simulink library "PM_BLDC"  (R2024a)
settings: Solver=VariableStepAuto  StartTime=0.0  StopTime=10.0  RelTol=1e-3
undefined symbols (not defined in the file): B, J, Ke, Ls, P, Rs
settings Model: Creator=Mohamed Draz  LastModifiedBy=Mohamed Draz

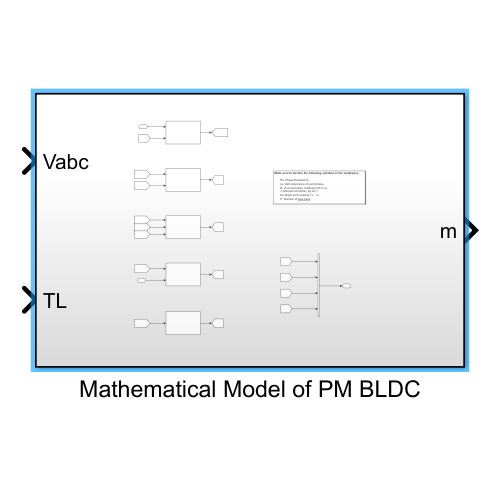
[thumbnail: Simulink's stored preview of the top-level diagram]
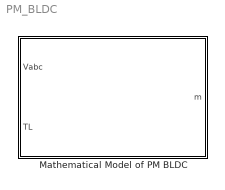
== system PM_BLDC ==
  Mathematical Model of PM BLDC : Subsystem

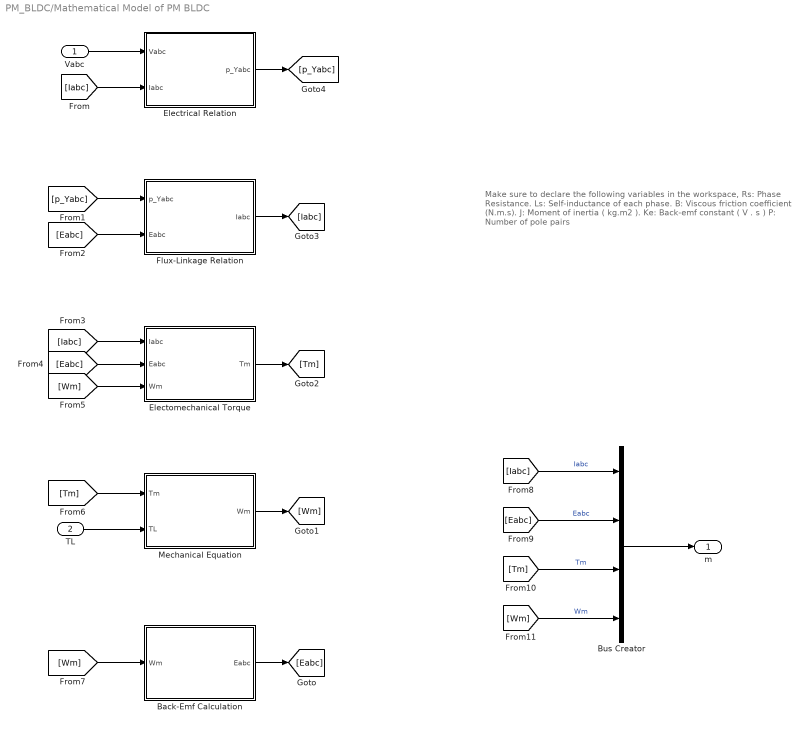
== system PM_BLDC/Mathematical Model of PM BLDC ==
  note: Make sure to declare the following variables in the workspace,
      |
      | Rs: Phase Resistance.
      | Ls: Self-inductance of each phase.
      | B: Viscous friction coefficient (N.m.s).
      | J: Moment of inertia ( kg.m2 ).
      | Ke: Back-emf constant ( V . s )
      | P: Number of pole pairs
  Vabc : Inport
  TL : Inport  Port=2
  Back-Emf Calculation : Subsystem
  Bus Creator : BusCreator  Inputs=4
  Electomechanical Torque : Subsystem
  Electrical Relation : Subsystem
  Flux-Linkage Relation : Subsystem
  Mechanical Equation : Subsystem
  m : Outport
  wires:
  [Wm] -> Back-Emf Calculation/1(Wm)
  [Eabc] -> Electomechanical Torque/2(Eabc)
  Electomechanical Torque/1(Tm) -> [Tm]
  Flux-Linkage Relation/1(Iabc) -> [Iabc]
  [Wm] -> Electomechanical Torque/3(Wm)
  [p_Yabc] -> Flux-Linkage Relation/1(p_Yabc)
  [Eabc] -> Flux-Linkage Relation/2(Eabc)
  [Iabc] -> Electomechanical Torque/1(Iabc)
  [Tm] -> Mechanical Equation/1(Tm)
  Back-Emf Calculation/1(Eabc) -> [Eabc]
  Vabc/1 -> Electrical Relation/1(Vabc)
  [Iabc] -> Electrical Relation/2(Iabc)
  TL/1 -> Mechanical Equation/2(TL)
  Electrical Relation/1(p_Yabc) -> [p_Yabc]
  Mechanical Equation/1(Wm) -> [Wm]
  [Iabc] -> Bus Creator/1  "Iabc"
  [Eabc] -> Bus Creator/2  "Eabc"
  [Tm] -> Bus Creator/3  "Tm"
  [Wm] -> Bus Creator/4  "Wm"
  Bus Creator/1 -> m/1

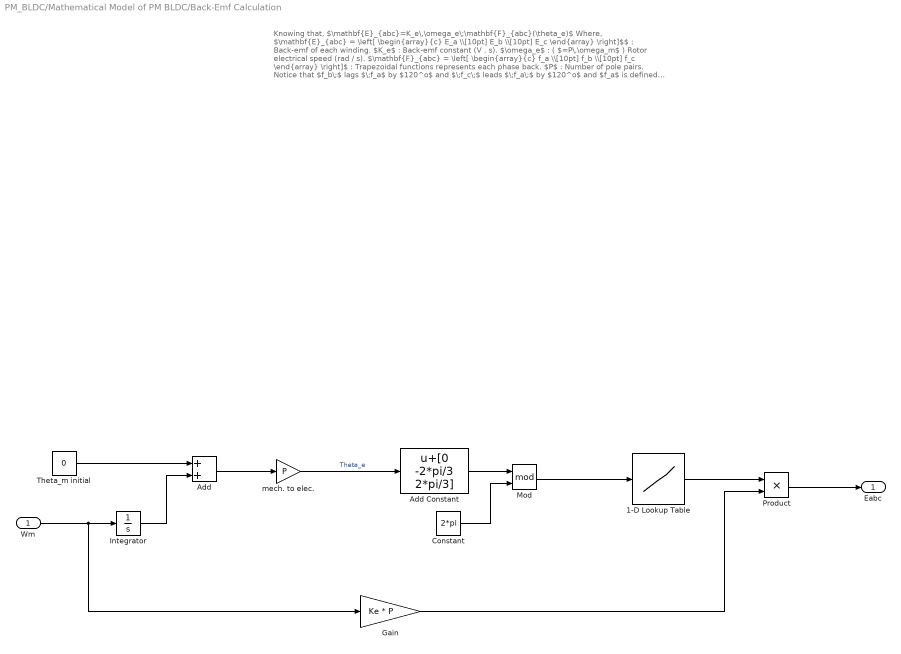
== system PM_BLDC/Mathematical Model of PM BLDC/Back-Emf Calculation ==
  note: Knowing that,
      |
      | $\mathbf{E}_{abc}=K_e\,\omega_e\;\mathbf{F}_{abc}(\theta_e)$
      |
      | Where,
      |
      | $\mathbf{E}_{abc} = \left[ \begin{array}{c} E_a \\[10pt] E_b \\[10pt] E_c \end{array} \right]$$ : Back-emf of each winding.
      |
      | $K_e$ : Back-emf constant (V . s).
      |
      | $\omega_e$ : ( $=P\,\omega_m$ ) Rotor electrical speed (rad / s).
      |
      | $\mathbf{F}_{abc} = \left[ \begin{array}{c} f_a \\[10pt] f_b \\[10pt] f_c \end{array} \right]$ : Trapezoidal functions represents each phase back.
      |
      | $P$ : Number of pole pairs.
      |
      | Notice that $f_b\;$ lags $\;f_a$ by $120^o$ and $\;f_c\;$ leads $\;f_a\;$ by $120^o$
      |
      | and $f_a$ is defined as,
      |
      | $f_a(\theta) = \begin{cases} 1 & 0 < \theta \le \frac{2\pi}{3} \\[6pt] 1 - \frac{6}{\pi}\left(\theta - \frac{2\pi}{3}\right) & \frac{2\pi}{3} < \theta \le \pi \\[6pt] -1 & \pi < \theta \le \frac{5\pi}{3} \\[6pt] -1 + \frac{6}{\pi}\left(\theta - \frac{5\pi}{3}\right) & \frac{5\pi}{3} < \theta \le 2\pi \end{cases}$$
  Wm : Inport
  1-D Lookup Table : Lookup_n-D  NumberOfTableDimensions=1  BreakpointsSpecification=Even spacing  BreakpointsForDimension1=[-5:5]  BreakpointsForDimension1FirstPoint=0  BreakpointsForDimension1Spacing=2*pi/6  Table=[1 1 1 -1 -1 -1 1]  InternalRulePriority=Speed  RndMeth=Simplest
  Add : Sum
  Add Constant : Bias  Bias=[0 -2*pi/3 2*pi/3]  SaturateOnIntegerOverflow=off
  Constant : Constant  Value=2*pi
  Gain : Gain  Gain=Ke * P
  Integrator : Integrator
  Mod : Math  Operator=mod
  Product : Product
  Theta_m initial : Constant  Value=0
  mech. to elec. : Gain  Gain=P
  Eabc : Outport
  wires:
  Add Constant/1 -> Mod/1
  Constant/1 -> Mod/2
  mech. to elec./1 -> Add Constant/1  "Theta_e"
  Theta_m initial/1 -> Add/1
  Mod/1 -> 1-D Lookup Table/1
  Gain/1 -> Product/2
  1-D Lookup Table/1 -> Product/1
  Wm/1 -> Gain/1, Integrator/1
  Product/1 -> Eabc/1
  Add/1 -> mech. to elec./1
  Integrator/1 -> Add/2

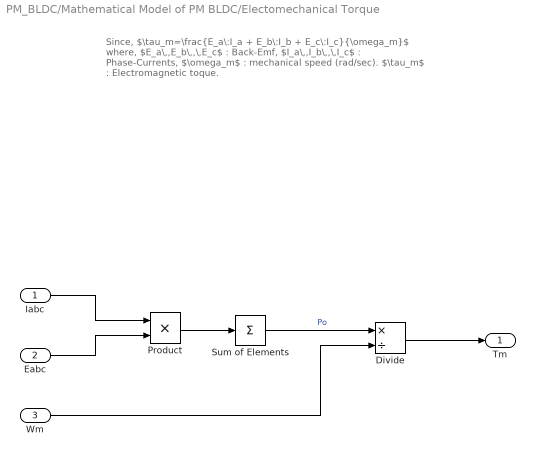
== system PM_BLDC/Mathematical Model of PM BLDC/Electomechanical Torque ==
  note: Since,
      |
      | $\tau_m=\frac{E_a\:I_a + E_b\:I_b + E_c\:I_c}{\omega_m}$
      |
      | where,
      |
      | $E_a\,,E_b\,,\,E_c$ : Back-Emf,
      | $I_a\,,I_b\,,\,I_c$ : Phase-Currents,
      | $\omega_m$ : mechanical speed (rad/sec).
      | $\tau_m$ : Electromagnetic toque.
  Iabc : Inport
  Eabc : Inport  Port=2
  Wm : Inport  Port=3
  Divide : Product  Inputs=*/
  Product : Product
  Sum of Elements : Sum  Inputs=+
  Tm : Outport
  wires:
  Sum of Elements/1 -> Divide/1  "Po"
  Wm/1 -> Divide/2
  Product/1 -> Sum of Elements/1
  Divide/1 -> Tm/1
  Iabc/1 -> Product/1
  Eabc/1 -> Product/2

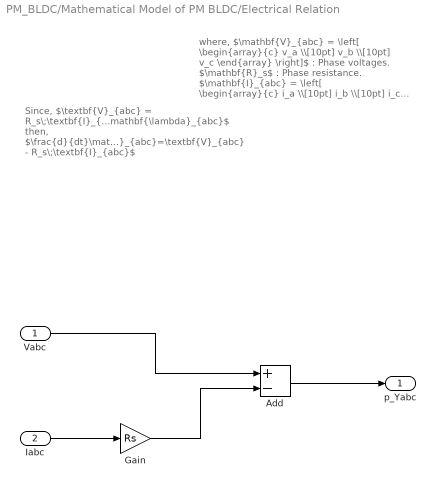
== system PM_BLDC/Mathematical Model of PM BLDC/Electrical Relation ==
  note: Since,
      | $\textbf{V}_{abc} = R_s\;\textbf{I}_{abc}+\frac{d}{dt}\mathbf{\lambda}_{abc}$
      |
      | then,
      | $\frac{d}{dt}\mathbf{\lambda}_{abc}=\textbf{V}_{abc} - R_s\;\textbf{I}_{abc}$
  note: where,
      | $\mathbf{V}_{abc} = \left[ \begin{array}{c} v_a \\[10pt] v_b \\[10pt] v_c \end{array} \right]$ : Phase voltages.
      |
      | $\mathbf{R}_s$ : Phase resistance.
      |
      | $\mathbf{I}_{abc} = \left[ \begin{array}{c} i_a \\[10pt] i_b \\[10pt] i_c \end{array} \right]$ Phase currents
      |
      | $\mathbf{\lambda}_{abc} = \left[ \begin{array}{c} \lambda_a \\[10pt] \lambda_b \\[10pt] \lambda_c \end{array} \right]$ Flux-linkages
  Vabc : Inport
  Iabc : Inport  Port=2
  Add : Sum  Inputs=+-
  Gain : Gain  Gain=Rs
  p_Yabc : Outport
  wires:
  Iabc/1 -> Gain/1
  Add/1 -> p_Yabc/1
  Gain/1 -> Add/2
  Vabc/1 -> Add/1

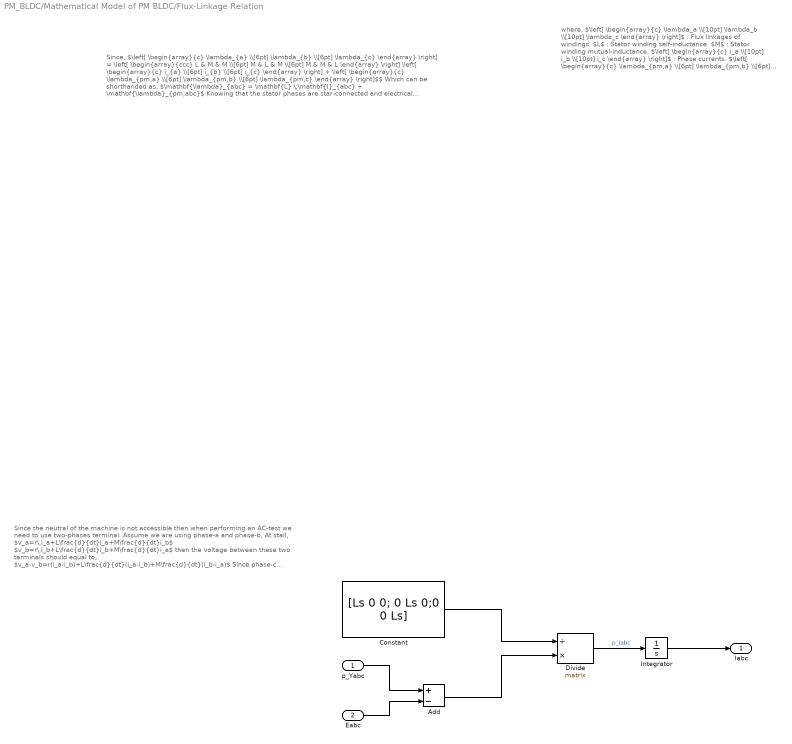
== system PM_BLDC/Mathematical Model of PM BLDC/Flux-Linkage Relation ==
  note: Since,
      |
      | $\left[ \begin{array}{c} \lambda_{a} \\[6pt] \lambda_{b} \\[6pt] \lambda_{c} \end{array} \right] = \left[ \begin{array}{ccc} L & M & M \\[6pt] M & L & M \\[6pt] M & M & L \end{array} \right] \left[ \begin{array}{c} i_{a} \\[6pt] i_{b} \\[6pt] i_{c} \end{array} \right] + \left[ \begin{array}{c} \lambda_{pm,a} \\[6pt] \lambda_{pm,b} \\[6pt] \lambda_{pm,c} \end{array} \right]$$
      |
      | Which can be shorthanded as,
      |
      | $\mathbf{\lambda}_{abc} = \mathbf{L} \;\mathbf{I}_{abc} + \mathbf{\lambda}_{pm,abc}$
      |
      | Knowing that the stator phases are star-connected and electrical parametes are assumed balanced,
      |
      | $i_a+i_b+i_c=0 \rightarrow i_b+i_c=-i_a$
      |
      | thus,
      | $\lambda_a=L\;i_a+M\;i_b+M\;i_c+\lambda_{pm,a}$
      |
      | turns into,
      | $\lambda_a=(L-M)\;i_a+\lambda_{pm,a}$
      |
      | The same could be done to windings b and c. So the original matrix turns into,
      |
      | $\left[ \begin{array}{c} \lambda_{a} \\[6pt] \lambda_{b} \\[6pt] \lambda_{c} \end{array} \right] = \left[ \begin{array}{ccc} L-M & 0 & 0 \\[6pt] 0 & L-M & 0 \\[6pt] 0 & 0 & L-M \end{array} \right] \left[ \begin{array}{c} i_{a} \\[6pt] i_{b} \\[6pt] i_{c} \end{array} \right] + \left[ \begin{array}{c} \lambda_{pm,a} \\[6pt] \lambda_{pm,b} \\[6pt] \lambda_{pm,c} \end{array} \right]$
      |
      | which can be short-handed as,
      |
      | $\mathbf{\lambda}_{abc} = \mathbf{L}_{new} \;\mathbf{I}_{abc} + \mathbf{\lambda}_{pm,abc}$
      |
      | Since $L$ and $M$ are both constants, taking the dervitave of both sides of equation results into,
      |
      | $\frac{d}{dt}\mathbf{\lambda}_{abc} = \mathbf{L}_{new} \;\frac{d}{dt}\mathbf{I}_{abc} + \frac{d}{dt}\mathbf{\lambda}_{pm,abc}$
      |
      | since $\frac{d}{dt}\mathbf{\lambda}_{pm,abc}$ is the the open-circuit voltage of each phase (i.e., Back-emf ) ,
      |
      | $\frac{d}{dt}\mathbf{\lambda}_{abc} = \mathbf{L}_{new} \;\frac{d}{dt}\mathbf{I}_{abc} + \mathbf{E}_{abc}$
      |
      | Finally,
      |
      | $\frac{d}{dt}\mathbf{I}_{abc} = \mathbf{L}_{new}^{-1} \;\left(\frac{d}{dt}\mathbf{\lambda}_{abc}-\mathbf{E}_{abc}\right)$
  note: where,
      |
      | $\left[ \begin{array}{c} \lambda_a \\[10pt] \lambda_b \\[10pt] \lambda_c \end{array} \right]$ : Flux linkages of windings.
      |
      | $L$ : Stator winding self-inductance.
      |
      | $M$ : Stator winding mutual-inductance.
      |
      | $\left[ \begin{array}{c} i_a \\[10pt] i_b \\[10pt] i_c \end{array} \right]$ : Phase currents.
      |
      | $\left[ \begin{array}{c} \lambda_{pm,a} \\[6pt] \lambda_{pm,b} \\[6pt] \lambda_{pm,c} \end{array} \right]$ : Flux-linkages caused by the permanent magent.
  note: Since the neutral of the machine is not accessible then when performing an AC-test we need to use two-phases terminal. Assume we are using phase-a and phase-b,
      |
      | At stall,
      |
      | $v_a=r\,i_a+L\frac{d}{dt}i_a+M\frac{d}{dt}i_b$
      | $v_b=r\,i_b+L\frac{d}{dt}i_b+M\frac{d}{dt}i_a$
      |
      | then the voltage between these two terminals should equal to,
      |
      | $v_a-v_b=r(i_a-i_b)+L\frac{d}{dt}(i_a-i_b)+M\frac{d}{dt}(i_b-i_a)$
      |
      | Since phase-c during this test is open-circuit. then, $i_a=-i_b=i$ . So,
      |
      | $v_a-v_b=2r\,i+2L\frac{d}{dt}i-2M\frac{d}{dt}i$
      | $v_a-v_b=2r\,i+2(L-M)\frac{d}{dt}i$
      |
      | this latest equation reveals that the inductance value measured between two phases during AC test is actually 2(L-M). So the phase-inductance value measured during AC-test mathimatically equals to (L-M).
      |
      | Finally,
      |
      | $L_s=L-M$
  p_Yabc : Inport
  Eabc : Inport  Port=2
  Add : Sum  Inputs=+-
  Constant : Constant  Value=[Ls 0 0; 0 Ls 0;0 0 Ls]  VectorParams1D=off
  Divide : Product  Inputs=/*  Multiplication=Matrix(*)
  Integrator : Integrator
  Iabc : Outport
  wires:
  Eabc/1 -> Add/2
  Divide/1 -> Integrator/1  "p_Iabc"
  p_Yabc/1 -> Add/1
  Integrator/1 -> Iabc/1
  Constant/1 -> Divide/1
  Add/1 -> Divide/2

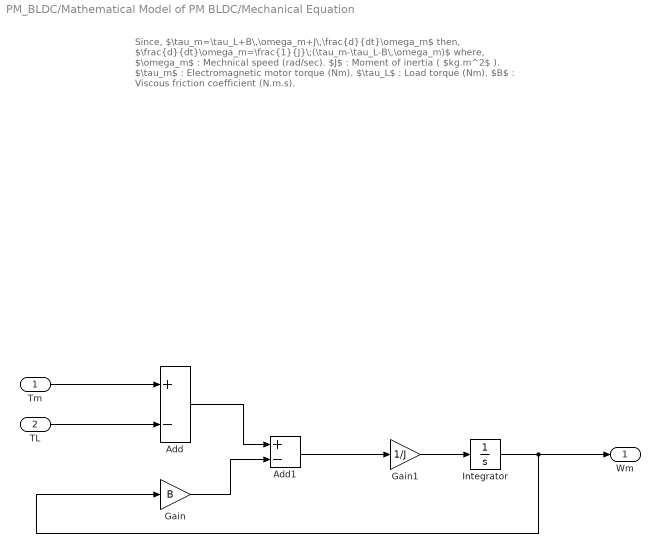
== system PM_BLDC/Mathematical Model of PM BLDC/Mechanical Equation ==
  note: Since,
      |
      | $\tau_m=\tau_L+B\,\omega_m+J\,\frac{d}{dt}\omega_m$
      |
      | then,
      |
      | $\frac{d}{dt}\omega_m=\frac{1}{J}\;(\tau_m-\tau_L-B\,\omega_m)$
      |
      | where,
      |
      | $\omega_m$ : Mechnical speed (rad/sec).
      | $J$ : Moment of inertia ( $kg.m^2$ ).
      | $\tau_m$ : Electromagnetic motor torque (Nm).
      | $\tau_L$ : Load torque (Nm).
      | $B$ : Viscous friction coefficient (N.m.s).
  Tm : Inport
  TL : Inport  Port=2
  Add : Sum  Inputs=+-
  Add1 : Sum  Inputs=+-
  Gain : Gain  Gain=B
  Gain1 : Gain  Gain=1/J
  Integrator : Integrator
  Wm : Outport
  wires:
  Gain/1 -> Add1/2
  Tm/1 -> Add/1
  Add1/1 -> Gain1/1
  Gain1/1 -> Integrator/1
  Integrator/1 -> Wm/1, Gain/1
  Add/1 -> Add1/1
  TL/1 -> Add/2
